simulink model "SIMULINK_REV0"  (R2020a)
settings: Solver=VariableStepAuto  StartTime=0.0  StopTime=0.2  RelTol=1e-3
values from neighbouring files (symbols this model uses):
  C = 7*Co_min_ripple    (= 0.000233333333333)    [Boost_Converter_Calc.m]    (also in TINH_TOAN_BO_DIEU_KHIEN_TYPE_III.m = 4.7e-05; boostControllerCalPID.m = 4.7e-05)
  Gc = kc*Gc1    [TINH_TOAN_BO_DIEU_KHIEN_TYPE_III.m]    (also in boostControllerCalPID.m)
  L = 0.9*Lmax    (= 1.3125e-05)    [Boost_Converter_Calc.m]    (also in TINH_TOAN_BO_DIEU_KHIEN_TYPE_III.m = 0.00012; boostControllerCalPID.m = 0.00012)
  R = Rmin    (= 15)    [Boost_Converter_Calc.m]    (also in TINH_TOAN_BO_DIEU_KHIEN_TYPE_III.m; boostControllerCalPID.m)
  Vg = 12    [TINH_TOAN_BO_DIEU_KHIEN_TYPE_III.m]    (also in boostControllerCalPID.m)
libraries: powerlib x11, powerlib_meascontrol x1
settings Model: Creator=ngtuan  LastModifiedBy=ngtuan
settings SolverCC: ZeroCrossAlgorithm=Adaptive
settings DebuggingCC: IgnoredZcDiagnostic=none

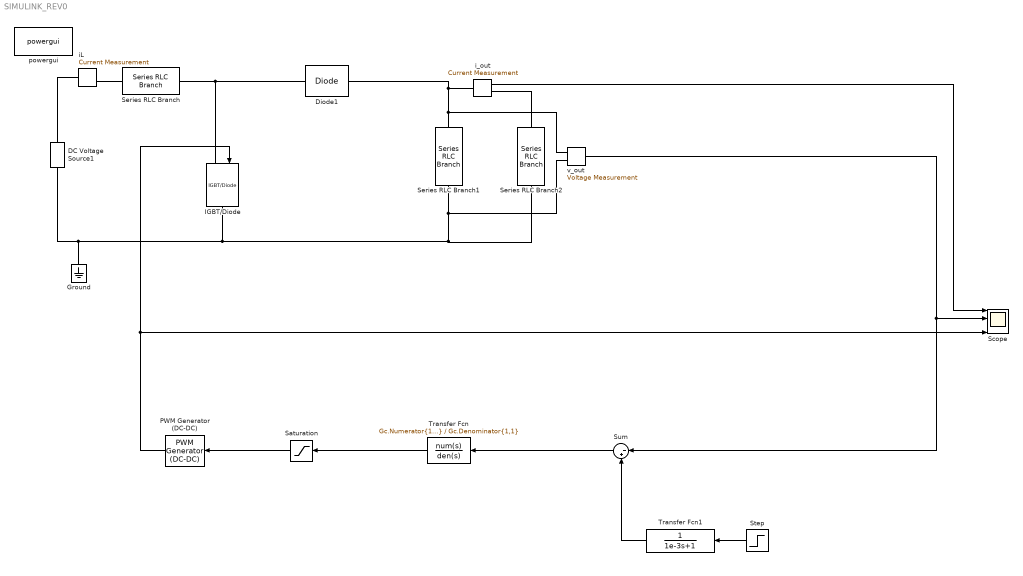
== system SIMULINK_REV0 ==
  DC Voltage Source1 : powerlib/Electrical Sources/DC Voltage Source  Amplitude=Vg  Measurements=None
  Diode1 : powerlib/Power Electronics/Diode  Ron=0.001  Lon=0  Vf=0  IC=0  UseSnubber=0  Rs=inf  Cs=inf  Measurements=off
  Ground : powerlib/Elements/Ground  LConnTagsString=a
  IGBT/Diode : powerlib/Power Electronics/IGBT//Diode  Ron=0.001  Rs=inf  Cs=inf  Measurements=off
  PWM Generator (DC-DC) : powerlib_meascontrol/Pulse & Signal Generators/PWM Generator (DC-DC)  Fsw=100000  Ts=0
  Saturation : Saturate  UpperLimit=1  LowerLimit=-1
  Scope : Scope  NumInputPorts=4
  Series RLC Branch : powerlib/Elements/Series RLC Branch  LConnTagsString=__new0  RConnTagsString=__new0  BranchType=L  Resistance=0  Inductance=L  SetiL0=off  InitialCurrent=0  Capacitance=0  Setx0=off  InitialVoltage=0  Measurements=None
  Series RLC Branch1 : powerlib/Elements/Series RLC Branch  LConnTagsString=__new0  RConnTagsString=__new0  BranchType=C  Resistance=70e-3  Inductance=1e-3  SetiL0=off  InitialCurrent=0  Capacitance=C  Setx0=on  InitialVoltage=12  Measurements=None
  Series RLC Branch2 : powerlib/Elements/Series RLC Branch  LConnTagsString=__new0  RConnTagsString=__new0  BranchType=R  Resistance=R  Inductance=1e-3  SetiL0=off  InitialCurrent=0  Capacitance=1000e-6  Setx0=off  InitialVoltage=0  Measurements=None
  Step : Step  Time=0.05  Before=20  After=30  SampleTime=0
  Sum : Sum  Inputs=|-+
  Transfer Fcn : TransferFcn  Numerator=Gc.Numerator{1,1}  Denominator=Gc.Denominator{1,1}
  Transfer Fcn1 : TransferFcn  Denominator=[1e-3 1]
  iL : powerlib/Measurements/Current Measurement  PhasorSimulation=off  OutputType=Complex  PSBequivalent=0
  i_out : powerlib/Measurements/Current Measurement  PhasorSimulation=off  OutputType=Complex  PSBequivalent=0
  powergui : powerlib/powergui  Priority=1  SimulationMode=Continuous  SampleTime=5e-6  frequency=60  Iterations=50  frequencyindice=0  Pbase=100e6  ErrMax=1e-4  UnitsV=kV  UnitsW=MW  buscounter=0  FunctionMessages=off  echomessages=off  EnableUseOfTLC=off  CurrentSourceSwitches=off  DisableSnubberDevices=off  DisableRonSwitches=off  DisableVfSwitches=off  DisplayEquations=off  AutomaticDiscreteSolvers=off  SolverType=Tustin/Backward Euler (TBE)  Interpol=off  ExternalGateDelay=off  methode=off  Ts=100  x0status=blocks  SPID=on  SwTol=0  HookPort=off  NonlinearTolerance=1e-4  nMaxIteration=100  ContinueOnMaxIteration=off  RestoreLinks=warning  ResistiveCurrentMeasurement=off  Frange=[0:2:500]  Ylog=off  Xlog=on  ShowGrid=off  save=off  variable=ZData  structure=0  ZoomFFT=off  StartTime=0.0  cycles=1  DisplayStyle=1  fundamental=60  FreqAxis=off  MaxFrequency=1000  frequencyindicesteady=1  RmsSteady=1  display=off
  v_out : powerlib/Measurements/Voltage Measurement  PhasorSimulation=off  OutputType=Complex  PSBequivalent=0
  wires:
  Transfer Fcn/1 -> Saturation/1
  i_out/1 -> Scope/1
  v_out/1 -> Sum/1, Scope/2
  PWM Generator (DC-DC)/1 -> Scope/4, IGBT/Diode/1
  Step/1 -> Transfer Fcn1/1
  Transfer Fcn1/1 -> Sum/2
  Sum/1 -> Transfer Fcn/1
  Saturation/1 -> PWM Generator (DC-DC)/1
  connections:
  DC Voltage Source1/LConn1 -- v_out/LConn2 -- Series RLC Branch1/RConn1 -- Series RLC Branch2/RConn1 -- IGBT/Diode/RConn1 -- Ground/LConn1
  i_out/LConn1 -- Diode1/RConn1 -- v_out/LConn1 -- Series RLC Branch1/LConn1
  i_out/RConn1 -- Series RLC Branch2/LConn1
  Series RLC Branch/RConn1 -- Diode1/LConn1 -- IGBT/Diode/LConn1
  iL/RConn1 -- Series RLC Branch/LConn1
  iL/LConn1 -- DC Voltage Source1/RConn1
